simulink model "rtwdemo_osek"  (Simulink 7.6)
settings: Solver=FixedStepDiscrete  StartTime=0.0  StopTime=10.0  RelTol=1e-3
PreLoadFcn:
  | addpath([matlabroot,'/toolbox/rtw/rtwdemos/osektgt_demo']);
  | mysig = Simulink.Signal;
  | mysig.RTWInfo.StorageClass = 'ExportedGlobal';
  | mysig.set('Description',...
  |   'ExportedGlobal signal - unstructured data',...
  |   'Min', 0, ...
  |   'Max',  3, ...
  |   'DocUnits',  'rpm');
PostLoadFcn:
  | if ~strcmp(computer,'PCWIN'), warndlg('This demo model can only be used on the 32-bit Windows platform.', 'Unsupported platform', 'modal'), end;
libraries: simulink x3, rtwdemowidgets x1
Description:
  | Interfacing to the OSEK Real-Time Operating System
CloseFcn:
  | rmpath([matlabroot,'/toolbox/rtw/rtwdemos/osektgt_demo']);
  | clear mysig
settings Model: Creator=The MathWorks Inc.  ExtModeAutoUpdateStatusClock=off
settings SolverCC: PositivePriorityOrder=on
settings DataIOCC: SaveOutput=off  SignalLogging=off  SaveTime=off  SignalLoggingName=sigsOut
settings OptimizationCC: InlineParams=on  InitFltsAndDblsToZero=on  EfficientMapNaN2IntZero=off  OptimizeModelRefInitCode=on  LifeSpan=1
settings DebuggingCC: SaveWithParameterizedLinksMsg=none  CheckExecutionContextPreStartOutputMsg=on  CheckExecutionContextRuntimeOutputMsg=on  SignalResolutionControl=TryResolveAllWithWarning  SolverPrmCheckMsg=none  MultiTaskDSMMsg=warning  MultiTaskCondExecSysMsg=none  StrictBusMsg=None
settings HardwareCC: ProdIntDivRoundTo=Zero  ProdEndianess=BigEndian  ProdHWDeviceType=Motorola PowerPC  TargetHWDeviceType=32-bit Generic
settings RTWCC: SystemTargetFile=ert.tlc  TLCOptions=-aRateBasedStepFcn=1  GenCodeOnly=on  GenerateMakefile=off  TemplateMakefile=ert_default_tmf  PostCodeGenCommand=osekPostCodeGenCommand  Description=Real-Time Workshop Embedded Coder (no auto configuration)  GenerateReport=on  RTWVerbose=off  ProcessScript=ert_make_rtw_hook  IncludeHyperlinkInReport=on  LaunchReport=on  IncludeERTFirstTime=on
settings CodeAppCC: IgnoreCustomStorageClasses=off  IgnoreTestpoints=on
settings ERTTargetCC: TargetFcnLib=ansi_tfl_tmw.mat  MultiwordLength=2048  ParenthesesLevel=Maximum  GenerateASAP2=on  InlinedParameterPlacement=NonHierarchical  ERTCustomFileTemplate=osek_file_process.tlc  ConvertIfToSwitch=off

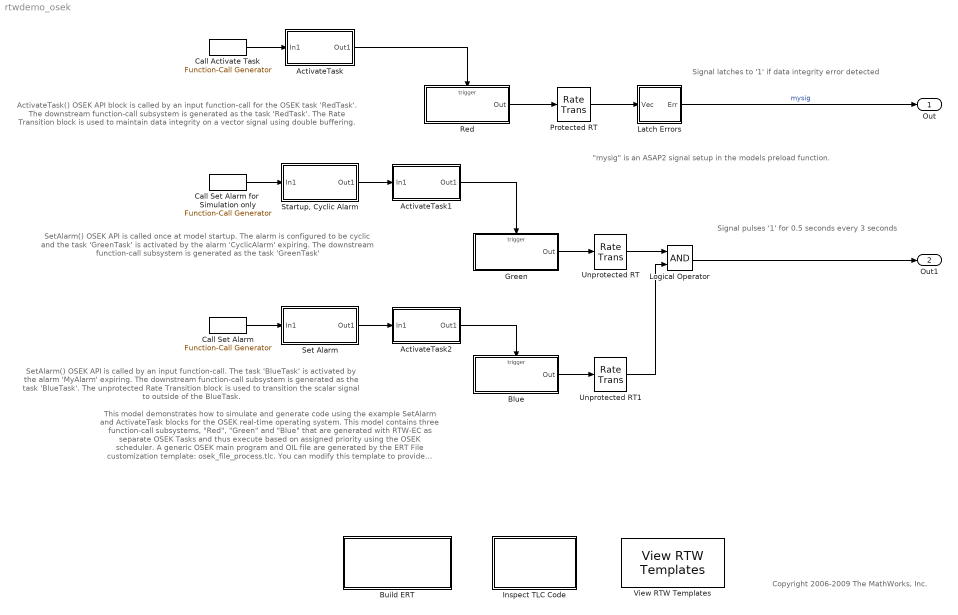
== system rtwdemo_osek ==
  note: This model demonstrates how to simulate and generate code using the example SetAlarm and ActivateTask blocks
      | for the OSEK real-time operating system. This model contains three function-call subsystems, "Red", "Green" and
      | "Blue" that are generated with RTW-EC as separate OSEK Tasks and thus execute based on assigned priority
      | using the OSEK scheduler. A generic OSEK main program and OIL file are generated by the ERT File customization
      | template: osek_file_process.tlc. You can modify this template to provide detailed information for your specific OSEK
      | implementation.
  note: ActivateTask() OSEK API block is called by an input
      | function-call for the OSEK task 'RedTask'. The downstream
      | function-call subsystem is generated as the task 'RedTask'.
      | The Rate Transition block is used to maintain data
      | integrity on a vector signal using double buffering.
  note: SetAlarm() OSEK API is called by an input function-call. The task
      | 'BlueTask' is activated by the alarm 'MyAlarm' expiring. The
      | downstream function-call subsystem is generated as the task 'BlueTask'.
      | The unprotected Rate Transition block is used to transition the
      | scalar signal to outside of the BlueTask.
  note: SetAlarm() OSEK API is called once at model startup. The alarm
      | is configured to be cyclic and the task 'GreenTask' is activated by
      | the alarm 'CyclicAlarm' expiring. The downstream function-call
      | subsystem is generated as the task 'GreenTask'
  note: Signal pulses '1' for 0.5 seconds every 3 seconds
  note: Signal latches to '1' if data integrity error detected
  note: "mysig" is an ASAP2 signal setup
      |  in the models preload function.
  note: Copyright 2006-2009 The MathWorks, Inc.
  ActivateTask : Subsystem  mask(OSEK Task Block){taskName=RedTask, taskPriority=10, taskStackSize=1000, taskSchedule=FULL}
      mask prompts: taskName "Task name (valid C identifier):"; taskPriority "Task priority (0-255):"; taskStackSize "Stack size (bytes):"; taskSchedule "Preemptive scheduling:"
      mask help: Defines the downstream function-call subsystem as an BCC1 OSEK task. The priority must be unique to the other tasks defined by the model.
      mask init:
      | if ~iscvar(taskName) & (length(taskName) > 0)
      |    errordlg('invalid Task Name, first character must be a letter or underscore and remaining characters must be letters,underscores or numbers.','Task Block Error','replace');
      |    taskName = '';
      | end
      mask Help: helpview([docroot '/toolbox/osek/osek.map'], 'osek_activatetask_blkref');
      mask StyleString: edit,edit,edit,popup(FULL|NON)
      mask Display:
      | disp(['       OSEK Task\n','       ''',taskName,''''])
      | port_label('input',1,'Call')
  ActivateTask1 : Subsystem  mask(OSEK Task Block){taskName=GreenTask, taskPriority=31, taskStackSize=100, taskSchedule=NON}
      mask prompts: taskName "Task name (valid C identifier):"; taskPriority "Task priority (0-255):"; taskStackSize "Stack size (bytes):"; taskSchedule "Preemptive scheduling:"
      mask help: Defines the downstream function-call subsystem as an BCC1 OSEK task. The priority must be unique to the other tasks defined by the model.
      mask init: same as rtwdemo_osek/ActivateTask
      mask Help: helpview([docroot '/toolbox/osek/osek.map'], 'osek_activatetask_blkref');
      mask StyleString: edit,edit,edit,popup(FULL|NON)
      mask Display:
      | disp(['       OSEK Task\n','       ''',taskName,''''])
      | port_label('input',1,'Call')
  ActivateTask2 : Subsystem  mask(OSEK Task Block){taskName=BlueTask, taskPriority=32, taskStackSize=100, taskSchedule=NON}
      mask prompts: taskName "Task name (valid C identifier):"; taskPriority "Task priority (0-255):"; taskStackSize "Stack size (bytes):"; taskSchedule "Preemptive scheduling:"
      mask help: Defines the downstream function-call subsystem as an BCC1 OSEK task. The priority must be unique to the other tasks defined by the model.
      mask init: same as rtwdemo_osek/ActivateTask
      mask Help: helpview([docroot '/toolbox/osek/osek.map'], 'osek_activatetask_blkref');
      mask StyleString: edit,edit,edit,popup(FULL|NON)
      mask Display:
      | disp(['       OSEK Task\n','       ''',taskName,''''])
      | port_label('input',1,'Call')
  Blue : Subsystem  TreatAsAtomicUnit=on
      settings: RTWSystemCode=Function
  Build ERT : Subsystem  mask{attrib_overrides={}}
      mask prompts: attrib_overrides "List of attributes to preserve (cell of strings):"
      mask help: Enter the attributes of the configuration set that you want preserved. Otherwise, the default configuration script will override your current settings.
      settings: OpenFcn=if ~strcmp(computer,'PCWIN'), warndlg('This demo model can only be used on the 32-bit Windows platform.', 'Unsupported platform', 'modal'), else, slbuild(bdroot), end;
      mask Display:
      | disp(['Generate Code Using\n',...
      | 	  'Real-Time Workshop\n',...
      | 	  'Embedded Coder\n'...
      | 	  '(double-click)'])
  Call Activate Task : simulink/Ports & Subsystems/Function-Call Generator  sample_time=.25  numberOfIterations=1
  Call Set Alarm : simulink/Ports & Subsystems/Function-Call Generator  sample_time=.75  numberOfIterations=1
  Call Set Alarm for  Simulation only : simulink/Ports & Subsystems/Function-Call Generator  sample_time=.5  numberOfIterations=1
  Green : Subsystem  TreatAsAtomicUnit=on
      settings: RTWSystemCode=Function
  Inspect TLC Code : Subsystem
      mask Display: disp('Inspect\nBlock\nTLC Code\n(double-click)')
  Latch Errors : Subsystem  TreatAsAtomicUnit=on
      settings: RTWSystemCode=Function
  Logical Operator : Logic  AllPortsSameDT=off  OutDataTypeStr=uint(8)
  Protected RT : RateTransition  Deterministic=off  OutPortSampleTime=1
  Red : Subsystem  TreatAsAtomicUnit=on
      settings: RTWSystemCode=Function
  Set Alarm : Subsystem  mask(OSEK Set Alarm Block){alarmName=MyAlarm, alarmIncr=1, alarmType=Relative, alarmPlacement=off, alarmCyclic=0}
      mask prompts: alarmName "Alarm name:"; alarmIncr "Increment:"; alarmType "Type:"; alarmPlacement "Call only at startup"; alarmCyclic "Cyclic:"
      mask help: Sets an OSEK alarm as specified. If 'Startup' placement is selected, the alarm is set only at model startup.
      mask init:
      | if ~iscvar(alarmName) & (length(alarmName) > 0)
      |    errordlg('invalid Alarm Name, first character must be a letter or underscore and remaining characters must be letters,underscores or numbers.','Task Block Error','replace');
      |    alarmName = '';
      | end
      mask Help: helpview([docroot '/toolbox/osek/osek.map'], 'osek_setalarm_blkref');
      mask StyleString: edit,edit,popup(Relative|Absolute),checkbox,edit
      mask CallbackString:
      | |||if strcmp(get_param(gcb,'alarmPlacement'),'on')
      | 	set_param(gcb,'MaskEnables', {'on', 'on', 'on', 'on', 'on'});
      | else
      | 	set_param(gcb,'MaskEnables', {'on', 'on', 'on', 'on', 'off'});
      | end
      | |
      mask Display:
      | disp(['         OSEK Alarm\n','       ''',alarmName,''''])
      | port_label('input',1,'Call')
  "Startup, Cyclic Alarm" : Subsystem  mask(OSEK Set Alarm Block){alarmName=cyclicAlarm, alarmIncr=1, alarmType=Relative, alarmPlacement=on, alarmCyclic=8}
      mask prompts: alarmName "Alarm name:"; alarmIncr "Increment:"; alarmType "Type:"; alarmPlacement "Call only at startup"; alarmCyclic "Cyclic:"
      mask help: Sets an OSEK alarm as specified. If 'Startup' placement is selected, the alarm is set only at model startup.
      mask init: same as rtwdemo_osek/Set Alarm
      mask Help: helpview([docroot '/toolbox/osek/osek.map'], 'osek_setalarm_blkref');
      mask StyleString: edit,edit,popup(Relative|Absolute),checkbox,edit
      mask CallbackString:
      | |||if strcmp(get_param(gcb,'alarmPlacement'),'on')
      | 	set_param(gcb,'MaskEnables', {'on', 'on', 'on', 'on', 'on'});
      | else
      | 	set_param(gcb,'MaskEnables', {'on', 'on', 'on', 'on', 'off'});
      | end
      | |
      mask Display:
      | disp(['         OSEK Alarm\n','       ''',alarmName,''''])
      | port_label('input',1,'Call')
  Unprotected RT : RateTransition  Integrity=off  OutPortSampleTime=.5
  Unprotected RT1 : RateTransition  Integrity=off  OutPortSampleTime=.5
  View RTW Templates : rtwdemowidgets/View RTW Templates  SystemSampleTime=-1
  Out : Outport
  Out1 : Outport  Port=2
  wires:
  ActivateTask/1(Out1) -> Red/Trigger
  Red/1(Out) -> Protected RT/1
  Call Activate Task/1 -> ActivateTask/1(In1)
  Latch Errors/1(Err) -> Out/1  "mysig"
  Protected RT/1 -> Latch Errors/1(Vec)
  Call Set Alarm/1 -> Set Alarm/1(In1)
  ActivateTask1/1(Out1) -> Green/Trigger
  Green/1(Out) -> Unprotected RT/1
  ActivateTask2/1(Out1) -> Blue/Trigger
  Blue/1(Out) -> Unprotected RT1/1
  Unprotected RT/1 -> Logical Operator/1
  Unprotected RT1/1 -> Logical Operator/2
  Logical Operator/1 -> Out1/1
  Call Set Alarm for  Simulation only/1 -> "Startup, Cyclic Alarm"/1(In1)
  Set Alarm/1(Out1) -> ActivateTask2/1(In1)
  "Startup, Cyclic Alarm"/1(Out1) -> ActivateTask1/1(In1)

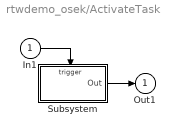
== system rtwdemo_osek/ActivateTask ==
  In1 : Inport
  Subsystem : Subsystem  TreatAsAtomicUnit=on
      settings: RTWSystemCode=Inline
  Out1 : Outport
  wires:
  Subsystem/1(Out) -> Out1/1
  In1/1 -> Subsystem/Trigger

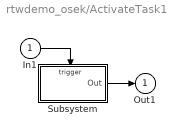
== system rtwdemo_osek/ActivateTask1 ==
  In1 : Inport
  Subsystem : Subsystem  TreatAsAtomicUnit=on
      settings: RTWSystemCode=Inline
  Out1 : Outport
  wires:
  Subsystem/1(Out) -> Out1/1
  In1/1 -> Subsystem/Trigger

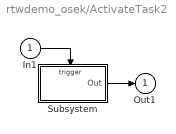
== system rtwdemo_osek/ActivateTask2 ==
  In1 : Inport
  Subsystem : Subsystem  TreatAsAtomicUnit=on
      settings: RTWSystemCode=Inline
  Out1 : Outport
  wires:
  Subsystem/1(Out) -> Out1/1
  In1/1 -> Subsystem/Trigger

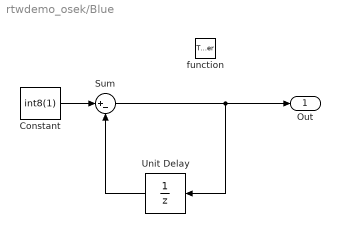
== system rtwdemo_osek/Blue ==
  function : TriggerPort  TriggerType=function-call
  Constant : Constant  Value=int8(1)
  Sum : Sum  Inputs=|+-  SaturateOnIntegerOverflow=on
  Unit Delay : UnitDelay  SampleTime=-1
  Out : Outport
  wires:
  Sum/1 -> Unit Delay/1, Out/1
  Constant/1 -> Sum/1
  Unit Delay/1 -> Sum/2

== system rtwdemo_osek/Build ERT ==

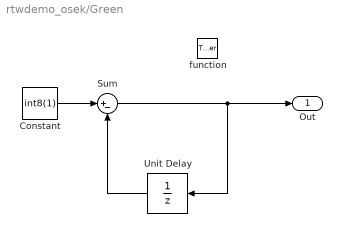
== system rtwdemo_osek/Green ==
  function : TriggerPort  TriggerType=function-call
  Constant : Constant  Value=int8(1)
  Sum : Sum  Inputs=|+-  SaturateOnIntegerOverflow=on
  Unit Delay : UnitDelay  SampleTime=-1
  Out : Outport
  wires:
  Unit Delay/1 -> Sum/2
  Constant/1 -> Sum/1
  Sum/1 -> Unit Delay/1, Out/1

== system rtwdemo_osek/Inspect TLC Code ==
  note: Real-Time Workshop uses the Target Language Compiler (TLC) as its final code generation stage.
      | TLC files are text based program files executed at the appropriate time by Real-Time Workshop.
      | Each block (type) has a corresponding TLC file, which allows easy modification or copying to create
      | additional OSEK OS API blocks.
  SubSystem11 : Subsystem
      settings: OpenFcn=edit(fullfile(matlabroot,'toolbox','rtw','rtwdemos','osektgt_demo','osektask.tlc'));
      mask Display: disp('Inspect\nActivateTask\nTLC File')
  SubSystem8 : Subsystem
      settings: OpenFcn=edit(fullfile(matlabroot,'toolbox','rtw','rtwdemos','osektgt_demo','oseksetalarm.tlc'));
      mask Display: disp('Inspect\nSetAlarm\nTLC File')

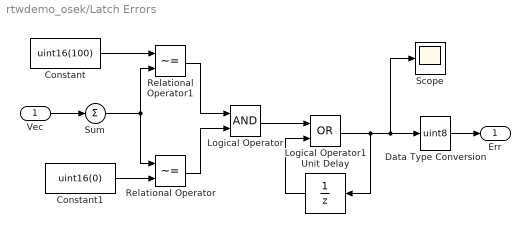
== system rtwdemo_osek/Latch Errors ==
  Vec : Inport
  Constant : Constant  Value=uint16(100)
  Constant1 : Constant  Value=uint16(0)
  Data Type Conversion : DataTypeConversion  OutDataTypeStr=uint8
  Logical Operator : Logic  AllPortsSameDT=off
  Logical Operator1 : Logic  Operator=OR  AllPortsSameDT=off
  Relational Operator : RelationalOperator  Operator=~=
  Relational Operator1 : RelationalOperator  Operator=~=
  Scope : Scope
  Sum : Sum  Inputs=1  SaturateOnIntegerOverflow=on
  Unit Delay : UnitDelay  SampleTime=-1
  Err : Outport
  wires:
  Vec/1 -> Sum/1
  Constant/1 -> Relational Operator1/1
  Constant1/1 -> Relational Operator/2
  Relational Operator1/1 -> Logical Operator/1
  Relational Operator/1 -> Logical Operator/2
  Logical Operator/1 -> Logical Operator1/1
  Logical Operator1/1 -> Unit Delay/1, Scope/1, Data Type Conversion/1
  Unit Delay/1 -> Logical Operator1/2
  Data Type Conversion/1 -> Err/1
  Sum/1 -> Relational Operator/1, Relational Operator1/2

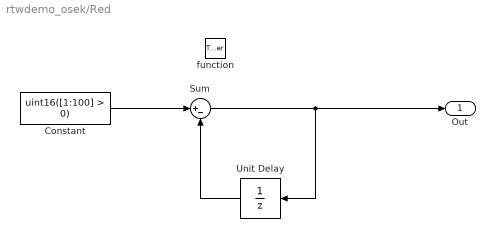
== system rtwdemo_osek/Red ==
  function : TriggerPort  TriggerType=function-call
  Constant : Constant  Value=uint16([1:100] > 0)  OutDataTypeStr=uint16
  Sum : Sum  Inputs=|+-  SaturateOnIntegerOverflow=on
  Unit Delay : UnitDelay  SampleTime=-1
  Out : Outport
  wires:
  Sum/1 -> Unit Delay/1, Out/1
  Constant/1 -> Sum/1
  Unit Delay/1 -> Sum/2

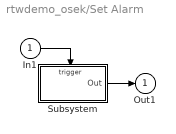
== system rtwdemo_osek/Set Alarm ==
  In1 : Inport
  Subsystem : Subsystem  TreatAsAtomicUnit=on
      settings: RTWSystemCode=Inline
      mask Type: VxWorks Task Block
  Out1 : Outport
  wires:
  In1/1 -> Subsystem/Trigger
  Subsystem/1(Out) -> Out1/1

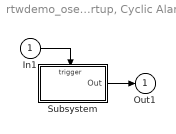
== system rtwdemo_osek/Startup, Cyclic Alarm ==
  In1 : Inport
  Subsystem : Subsystem  TreatAsAtomicUnit=on
      settings: RTWSystemCode=Inline
      mask Type: VxWorks Task Block
  Out1 : Outport
  wires:
  In1/1 -> Subsystem/Trigger
  Subsystem/1(Out) -> Out1/1

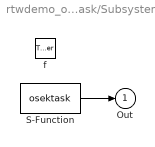
== system rtwdemo_osek/ActivateTask/Subsystem ==
  f : TriggerPort  TriggerType=function-call
  S-Function : S-Function  FunctionName=osektask  Parameters=taskName, taskPriority, taskStackSize, taskSchedule  EnableBusSupport=off
  Out : Outport
  wires:
  S-Function/1 -> Out/1

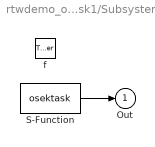
== system rtwdemo_osek/ActivateTask1/Subsystem ==
  f : TriggerPort  TriggerType=function-call
  S-Function : S-Function  FunctionName=osektask  Parameters=taskName, taskPriority, taskStackSize, taskSchedule  EnableBusSupport=off
  Out : Outport
  wires:
  S-Function/1 -> Out/1

== system rtwdemo_osek/ActivateTask2/Subsystem ==
  f : TriggerPort  TriggerType=function-call
  S-Function : S-Function  FunctionName=osektask  Parameters=taskName, taskPriority, taskStackSize, taskSchedule  EnableBusSupport=off
  Out : Outport
  wires:
  S-Function/1 -> Out/1

== system rtwdemo_osek/Inspect TLC Code/SubSystem11 ==

== system rtwdemo_osek/Inspect TLC Code/SubSystem8 ==

== system rtwdemo_osek/Set Alarm/Subsystem ==
  f : TriggerPort  TriggerType=function-call
  S-Function : S-Function  FunctionName=oseksetalarm  Parameters=alarmName, alarmIncr, alarmCyclic, alarmType, alarmPlacement  EnableBusSupport=off
  Out : Outport
  wires:
  S-Function/1 -> Out/1

== system rtwdemo_osek/Startup, Cyclic Alarm/Subsystem ==
  f : TriggerPort  TriggerType=function-call
  S-Function : S-Function  FunctionName=oseksetalarm  Parameters=alarmName, alarmIncr, alarmCyclic, alarmType, alarmPlacement  EnableBusSupport=off
  Out : Outport
  wires:
  S-Function/1 -> Out/1
